simulink library "WBToolboxLibrary"  (R2014b)
settings: Solver=ode45  StartTime=0.0  StopTime=10.0  RelTol=1e-3
undefined symbols (not defined in the file): WBT_modelName, WBT_robotName, WBT_wbiFilename, WBT_wbiList
libraries: simulink x1
(part 1 of 2)
settings Model: CovSaveCumulativeToWorkspaceVar=on  Creator=jorhabib  LastModifiedBy=csartore

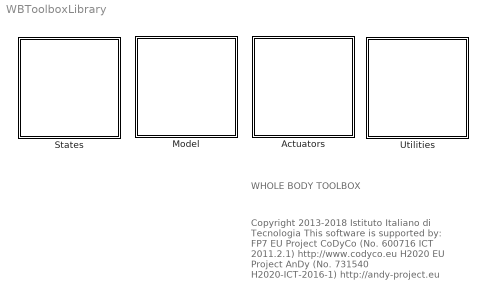
== system WBToolboxLibrary ==
  note: WHOLE BODY TOOLBOX
  note: Copyright 2013-2018 Istituto Italiano di Tecnologia
      |
      | This software is supported by:
      | FP7 EU Project CoDyCo (No. 600716 ICT 2011.2.1) http://www.codyco.eu
      | H2020 EU Project AnDy (No. 731540 H2020-ICT-2016-1) http://andy-project.eu
  Actuators : Subsystem
      mask Display: image(imread('wholeBodyActuators.png'),'center')
  Model : Subsystem
      mask Display: image(imread('wholeBodyModel.png'),'center')
  States : Subsystem
      mask Display: image(imread('wholeBodyStates.png'),'center');
  Utilities : Subsystem
      mask Display: image(imread('utilities.png'))

== system WBToolboxLibrary/Actuators ==
  SetMotorParameters : S-Function  FunctionName=BlockFactory  Parameters='SetMotorParameters','WBToolbox',WBTConfigParameters,configBlockAbsName,readP,readI,readD,pidType,setKTau,kTau,setBemf,bemf  SFunctionDeploymentMode=off  EnableBusSupport=off  mask(SetMotorParameters){pidType=Position, readP=on, readI=off, readD=off, setKTau=off, kTau=[0], setBemf=off, bemf=[0]}
      mask prompts: pidType "PID Type"; readP "Enable P gains input signal"; readI "Enable I gains input signal"; readD "Enable D gains input signal"; setKTau "Set motor constant KTau"; setBemf "Set motor back EMF constant"
      mask help:
      | This block allows to set motor PIDs and constants such as the motor constant and the back EMF.
      |
      | The motor constant and the back EMF are set in the block's mask, and their values are applied during the first simulation loop. The PIDs values are instead set from the input ports.
      |
      | All these vectors should have a size equal to the number of controlled joints specified in the referred Configuration block.
      |
      | At the end of the simulation, the default values are restored.
      mask init:
      | % WBBlock Initialization
      | % ======================
      | 
      | try
      |     [configBlockAbsName, WBTConfig] = WBToolbox.BlockInitialization(gcb, gcs);
      |     
      |     WBTConfigParameters = WBTConfig.getSimulinkParameters;
      |     clear WBTConfig;
      | catch
      | end
      | 
      | % The booleans of the checkboxes always create problems
      | readP = uint8(readP);
      | readI = uint8(readI);
      | readD = uint8(readD);
      mask TypeOptions pidType: Position | Torque
      mask Callback pidType:
      | % Get the mask parameter values. This is a cell
      | %   array of strings.
      | maskStr = get_param(gcb,'pidType');
      | 
      | switch maskStr
      |     case 'Position'
      |         set_param(gcb,'BackgroundColor', '[0.5137, 0.8510, 0.6706, 1.0]');
      |     case 'Position Direct'
      |         set_param(gcb,'BackgroundColor', '[0.3922, 0.7882, 0.3451, 1.0]');
      |     case 'Velocity'
      |         set_param(gcb,'BackgroundColor', '[0.5137, 0.6745, 1.0000, 1.0]');
      |     case 'Torque'
      |         set_param(gcb,'BackgroundColor', '[0.8275, 0.5765, 0.6039, 1.0]');
      |     otherwise
      |         error('PID Type not recognized');
      | end
      | 
      | clear  maskStr
      mask Callback setKTau:
      | h = Simulink.Mask.get(gcb);
      | setKTauValue = get_param(gcb,'setKTau');
      | 
      | if ~strcmp(setKTauValue,'on')
      |     h.Parameters(6).Enabled = 'off';
      | else
      |     h.Parameters(6).Enabled = 'on';
      | end
      | 
      | clear h setKTauValue
      mask Callback setBemf:
      | h = Simulink.Mask.get(gcb);
      | setBemfValue = get_param(gcb,'setBemf');
      | 
      | if ~strcmp(setBemfValue,'on')
      |     h.Parameters(8).Enabled = 'off';
      | else
      |     h.Parameters(8).Enabled = 'on';
      | end
      | 
      | clear h setBemfValue
      mask DialogControl Control2 Prompt: Toggle Config Block Highlighting
      mask DialogControl Control2 Callback:
      | [configBlock, ~] = WBToolbox.BlockInitialization(gcb, gcs);
      | 
      | try
      |     if (strcmp(get_param(configBlock,'HiliteAncestors'),'none'))
      |         hilite_system(configBlock,'find');
      |     else
      |         hilite_system(configBlock,'none');
      |     end
      | catch
      |     error('[%s:ShowConfigBlock:Callback] Failed to process config block name: %s',gcb,configBlock);
      | end
      | 
      | clear configBlock
      mask Display:
      | fprintf('Motor Parameters\n(%s)',pidType);
      | 
      | numPorts = 0;
      | 
      | if readP
      |     numPorts = numPorts + 1;
      |     port_label('input',numPorts,'P')
      | end
      | 
      | if readI
      |     numPorts = numPorts + 1;
      |     port_label('input',numPorts,'I')
      | end
      | 
      | if readD
      |     numPorts = numPorts + 1;
      |     port_label('input',numPorts,'D')
      | end
  SetMotorReferences : Subsystem  mask(SetMotorReferences){controlType=Current}
      mask prompts: controlType "Control Mode"
      mask help:
      | This block sets motor references. The type of control mode is specified as a parameter in the block.
      |
      | Assuming N as the number of motors (usually equal to internal DoFs):
      |
      | Input:
      |   - References: Vector of size N, representing the references to be sent to the robot controlled motors.
      |
      | Parameters:
      |   - Control Mode: The control mode. Choose one of the supplied mode.
      |
      | Unit of measurement:
      |   - PWM  [-100, 100]% Duty cycle
      |   - Current [A]
      |   - Back EMF
      |   - Torque Constant
      mask init:
      | refSpeed = 0;
      | 
      | % WBBlock Initialization
      | % ======================
      | 
      | try
      |     [configBlockAbsName, WBTConfig] = WBToolbox.BlockInitialization(gcb, gcs);
      |     
      |     WBTConfigParameters = WBTConfig.getSimulinkParameters;
      |     clear WBTConfig;
      | catch
      | end
      mask TypeOptions controlType: PWM | Current | Back EMF | Torque Constant
      mask Callback controlType:
      | % Get the mask parameter values. This is a cell
      | %   array of strings.
      | 
      | maskStr = get_param(gcb,'controlType');
      | 
      | switch maskStr
      |     case 'PWM'
      |         set_param(gcb,'BackgroundColor', '[1, 1, 1, 1.0]');
      |     case 'Current'
      |         set_param(gcb,'BackgroundColor', '[0.96, 0.77, 0.46, 1.0]');
      |     case 'Back EMF'
      |         set_param(gcb,'BackgroundColor', '[0.8, 0.4, 1.0, 1.0]');
      |     case 'Torque Constant'
      |         set_param(gcb,'BackgroundColor', '[0.8, 1.0, 0.4, 1.0]');
      |     otherwise
      |         error('Control Type not recognized.')
      | end
      | 
      | clear  maskStr
      mask DialogControl toggleHighlighting Prompt: Toggle Config Block Highlighting
      mask DialogControl toggleHighlighting Callback:
      | [configBlock, ~] = WBToolbox.BlockInitialization(gcb, gcs);
      | 
      | try
      |     if (strcmp(get_param(configBlock,'HiliteAncestors'),'none'))
      |         hilite_system(configBlock,'find');
      |     else
      |         hilite_system(configBlock,'none');
      |     end
      | catch
      |     error('[%s:ShowConfigBlock:Callback] Failed to process config block name: %s',gcb,configBlock);
      | end
      | 
      | clear configBlock
      mask Display:
      | disp(get_param(gcb,'controlType'))
      | %port_label('input',1,'References')
  SetReferences : Subsystem  mask(SetReferences){controlType=Position, refSpeed=10*(pi/180), refAcceleration=1000000*(pi/180)}
      mask prompts: controlType "Control Mode"; refSpeed "Reference Speed"; refAcceleration "Reference Velocity"
      mask help:
      | This block sets the references for the robot actuators.
      | The type of control mode is specified as a parameter in the block.
      |
      | Assuming DoFs is the number of internal degrees of freedom configured in the associated Config block:
      |
      | Input:
      |   - References: Vector of size DoFs, representing the references to be sent to the robot controlled joints.
      |   - Reference Speed (Position): Set the reference speed in rad/s used by the trajectory generator of the IPositionControl interface
      |   - Reference Acceleration (Velocity): Set the reference speed in rad/s/s used by the trajectory generator of the IVelocityControl interface
      |
      | Parameters:
      |   - Control Mode: The control mode. Choose one of the supplied mode.
      |
      | Unit of measurement:
      | - Position [rad]
      | - Velocity [rad/s]
      | - Acceleration [rad/s/s]
      | - Torque [Nm]
      mask init:
      | if (strcmp(controlType,'Position'))
      |     refTrajectory = refSpeed;
      | elseif (strcmp(controlType,'Velocity'))
      |     refTrajectory = refAcceleration;
      | else
      |     refTrajectory = 0;
      | end
      | 
      | % WBBlock Initialization
      | % ======================
      | 
      | try
      |     [configBlockAbsName, WBTConfig] = WBToolbox.BlockInitialization(gcb, gcs);
      |     
      |     WBTConfigParameters = WBTConfig.getSimulinkParameters;
      |     clear WBTConfig;
      | catch
      | end
      mask TypeOptions controlType: Position | Position Direct | Velocity | Torque
      mask Callback controlType:
      | % Get the mask parameter values. This is a cell
      | %   array of strings.
      | 
      | maskStr = get_param(gcb,'controlType');
      | 
      | switch maskStr
      |     case 'Position'
      |         set_param(gcb,'BackgroundColor', '[0.5137, 0.8510, 0.6706, 1.0]');
      |         set_param(gcb,'MaskVisibilities', {'on';'on';'off'});
      |     case 'Position Direct'
      |         set_param(gcb,'BackgroundColor', '[0.3922, 0.7882, 0.3451, 1.0]');
      |         set_param(gcb,'MaskVisibilities', {'on';'off';'off'});
      |     case 'Velocity'
      |         set_param(gcb,'BackgroundColor', '[0.5137, 0.6745, 1.0000, 1.0]');
      |         set_param(gcb,'MaskVisibilities', {'on';'off';'on'});
      |     case 'Torque'
      |         set_param(gcb,'BackgroundColor', '[0.8275, 0.5765, 0.6039, 1.0]');
      |         set_param(gcb,'MaskVisibilities', {'on';'off';'off'});
      |     otherwise
      |         error('Control Type not recognized.')
      | end
      | 
      | clear  maskStr
      mask DialogControl toggleHighlighting Prompt: Toggle Config Block Highlighting
      mask DialogControl toggleHighlighting Callback:
      | [configBlock, ~] = WBToolbox.BlockInitialization(gcb, gcs);
      | 
      | try
      |     if (strcmp(get_param(configBlock,'HiliteAncestors'),'none'))
      |         hilite_system(configBlock,'find');
      |     else
      |         hilite_system(configBlock,'none');
      |     end
      | catch
      |     error('[%s:ShowConfigBlock:Callback] Failed to process config block name: %s',gcb,configBlock);
      | end
      | 
      | clear configBlock
      mask Display:
      | disp(get_param(gcb,'controlType'))
      | %port_label('input',1,'References')

== system WBToolboxLibrary/Model ==
  Dynamics : Subsystem
      mask Display: image(imread('Dynamics.png'))
  Jacobians : Subsystem
      mask Display: image(imread('jacobian.png'))
  Kinematics : Subsystem
      mask Display: image(imread('forwardKinematics.png'))

== system WBToolboxLibrary/States ==
  GetLimits : Subsystem  mask(GetLimits){limitsSource=ControlBoard, limitsType=Position}
      mask prompts: limitsSource "Limits Source"; limitsType "Limits Type"
      mask help:
      | This block provides the joint limits gathering data from either the Robot's Control Board or URDF model.
      |
      | Output:
      |   - Max: 1xDoFs vector containing the maximum limit
      |   - Min:  1xDoFs vector containing the maximum limit
      |
      | Unit of measurement:
      |   - Position: rad
      |   - Velocity: rad/sec
      mask init:
      | % WBBlock Initialization
      | % ======================
      | 
      | try
      |     [configBlockAbsName, WBTConfig] = WBToolbox.BlockInitialization(gcb, gcs);
      |     
      |     WBTConfigParameters = WBTConfig.getSimulinkParameters;
      |     clear WBTConfig;
      | catch
      | end
      | 
      | % GetLimits Initialization
      | % =========================
      | 
      | sourceLimit = get_param(gcb,'limitsSource');
      | typeLimit = get_param(gcb,'limitsType');
      | notifyError = false;
      | 
      | switch sourceLimit
      |     case 'ControlBoard'
      |         switch typeLimit
      |             case 'Position'
      |                 limitsType = 'ControlBoardPosition';
      |             case 'Velocity'
      |                 limitsType = 'ControlBoardVelocity';
      |             otherwise
      |                 notifyError = true;
      |         end
      |     case 'URDF'
      |         switch typeLimit
      |             case 'Position'
      |                 limitsType = 'ModelPosition';
      |             otherwise
      |                 notifyError = true;
      |         end
      | end
      | 
      | if notifyError
      |     error('Limit Type not recognized');
      | end
      | 
      | clear sourceLimit typeLimit notifyError
      mask TypeOptions limitsSource: ControlBoard | URDF
      mask Callback limitsSource:
      | sourceLimit = get_param(gcb,'limitsSource');
      | blockParameters = Simulink.Mask.get(gcb).Parameters;
      | limitsTypeBlockParam = blockParameters(2);
      | 
      | switch sourceLimit
      |     case 'ControlBoard'
      |         limitsTypeBlockParam.TypeOptions = {'Position','Velocity'};
      |         %limitsTypeBlockParam.Value = limitsTypeBlockParam.TypeOptions{1};
      |     case 'URDF'
      |         limitsTypeBlockParam.TypeOptions = {'Position'};
      |         %limitsTypeBlockParam.Value = limitsTypeBlockParam.TypeOptions{1};
      |     otherwise
      |         error('Limit Source not recognized');
      | end
      | 
      | clear sourceLimit blockParameters limitsTypeBlockParam
      mask TypeOptions limitsType: Position | Velocity
      mask Callback limitsType:
      | % Get the mask parameter values. This is a cell array of strings.
      | %
      | maskStr = get_param(gcb,'limitsType');
      | if strcmp(maskStr, 'Position')
      |     set_param(gcb,'BackgroundColor', '[0.5137, 0.8510, 0.6706, 1.0]');
      | elseif strcmp(maskStr, 'Velocity')
      |     set_param(gcb,'BackgroundColor', '[0.5137, 0.6745, 1.0000, 1.0]');
      | elseif strcmp(maskStr, 'Acceleration')
      |     set_param(gcb,'BackgroundColor', '[0.9255, 0.8706, 0.1333, 1.0]');
      | elseif strcmp(maskStr, 'Torque')
      |     set_param(gcb,'BackgroundColor', '[0.8275, 0.5765, 0.6039, 1.0]');
      | end
      | clear  maskStr
      mask DialogControl toggleHighlighting Prompt: Toggle Config Block Highlighting
      mask DialogControl toggleHighlighting Callback:
      | [configBlock, ~] = WBToolbox.BlockInitialization(gcb, gcs);
      | 
      | try
      |     if (strcmp(get_param(configBlock,'HiliteAncestors'),'none'))
      |         hilite_system(configBlock,'find');
      |     else
      |         hilite_system(configBlock,'none');
      |     end
      | catch
      |     error('[%s:ShowConfigBlock:Callback] Failed to process config block name: %s',gcb,configBlock);
      | end
      | 
      | clear configBlock
      mask Display:
      | fprintf('%s\n(%s)',get_param(gcb,'limitsType'),get_param(gcb,'limitsSource'))
      | 
      | port_label('output',1,'Min')
      | port_label('output',2,'Max')
  GetMeasurement : Subsystem  mask(GetMeasurement){measuredType=Joints Position}
      mask prompts: measuredType "Estimate Type"
      mask help:
      | This block gathers the measurement of the specified type.
      |
      | Assuming DoFs is the number of degrees of freedom of the robot,
      |
      | Output:
      |   - References: Vector of size DoFs, representing the requested measurement.
      |
      | Parameters:
      |   - Control Mode: The control mode. Choose one of the supplied mode.
      |
      | Unit of measurement:
      |   - Position: rad
      |   - Velocity: rad/sec
      |   - Acceleration: rad/sec/sec
      |   - Torque: Nm
      mask init:
      | % WBBlock Initialization
      | % ======================
      | 
      | try
      |     [configBlockAbsName, WBTConfig] = WBToolbox.BlockInitialization(gcb, gcs);
      |     
      |     WBTConfigParameters = WBTConfig.getSimulinkParameters;
      |     clear WBTConfig;
      | catch
      | end
      mask TypeOptions measuredType: Joints Position | Joints Velocity | Joints Acceleration | Joints Torque
      mask Callback measuredType:
      | % Get the mask parameter values. This is a cell
      | %   array of strings.
      | 
      | maskStr = get_param(gcb,'measuredType');
      | if strcmp(maskStr, 'Joints Position')
      |     set_param(gcb,'BackgroundColor', '[0.5137, 0.8510, 0.6706, 1.0]');
      | elseif strcmp(maskStr, 'Joints Velocity')
      |     set_param(gcb,'BackgroundColor', '[0.5137, 0.6745, 1.0000, 1.0]');
      | elseif strcmp(maskStr, 'Joints Acceleration')
      |     set_param(gcb,'BackgroundColor', '[0.9255, 0.8706, 0.1333, 1.0]');
      | elseif strcmp(maskStr, 'Joints Torque')
      |     set_param(gcb,'BackgroundColor', '[0.8275, 0.5765, 0.6039, 1.0]');
      | end
      | clear  maskStr
      mask DialogControl toggleHighlighting Prompt: Toggle Config Block Highlighting
      mask DialogControl toggleHighlighting Callback:
      | [configBlock, ~] = WBToolbox.BlockInitialization(gcb, gcs);
      | 
      | try
      |     if (strcmp(get_param(configBlock,'HiliteAncestors'),'none'))
      |         hilite_system(configBlock,'find');
      |     else
      |         hilite_system(configBlock,'none');
      |     end
      | catch
      |     error('[%s:ShowConfigBlock:Callback] Failed to process config block name: %s',gcb,configBlock);
      | end
      | 
      | clear configBlock
      mask Display: port_label('output', 1, get_param(gcb,'measuredType'))
  GetMotorMeasurement : Subsystem  mask(GetMeasurement){measuredType=Motor Current}
      mask prompts: measuredType "Estimate Type"
      mask help:
      | This block gathers the measurement of the specified type.
      |
      | Assuming DoFs is the number of degrees of freedom of the robot,
      |
      | Output:
      |   - References: Vector of size DoFs, representing the requested measurement.
      |
      | Parameters:
      |   - Control Mode: The control mode. Choose one of the supplied mode.
      |
      | Unit of measurement:
      |   - PWM: duty cycle expressed as percentage [-100, 100]%
      |   - Current: values in Ampere
      mask init: same as WBToolboxLibrary/States/GetMeasurement
      mask TypeOptions measuredType: Motor Position | Motor Velocity | Motor Acceleration | Motor PWM | Motor Current | Motor Back EMF | Motor Torque Constant
      mask Callback measuredType:
      | maskStr = get_param(gcb,'measuredType');
      | 
      | switch maskStr
      |     case 'Motor Position'
      |         set_param(gcb,'BackgroundColor', '[0.5137, 0.8510, 0.6706, 1.0]');
      |     case 'Motor Velocity'
      |         set_param(gcb,'BackgroundColor', '[0.5137, 0.6745, 1.0000, 1.0]');
      |     case 'Motor Acceleration'
      |         set_param(gcb,'BackgroundColor', '[0.9255, 0.8706, 0.1333, 1.0]');
      |     case 'Motor PWM'
      |         set_param(gcb,'BackgroundColor', '[1, 1, 1, 1.0]');
      |     case 'Motor Current'
      |         set_param(gcb,'BackgroundColor', '[0.96, 0.77, 0.46, 1.0]');
      |     case 'Motor Back EMF'
      |         set_param(gcb,'BackgroundColor', '[0.8, 0.4, 1.0, 1.0]');
      |     case 'Motor Torque Constant'
      |         set_param(gcb,'BackgroundColor', '[0.8, 1.0, 0.4, 1.0]');
      |     otherwise
      |         error('Control Type not recognized.')
      | end
      | 
      | clear maskStr
      mask DialogControl toggleHighlighting Prompt: Toggle Config Block Highlighting
      mask DialogControl toggleHighlighting Callback:
      | [configBlock, ~] = WBToolbox.BlockInitialization(gcb, gcs);
      | 
      | try
      |     if (strcmp(get_param(configBlock,'HiliteAncestors'),'none'))
      |         hilite_system(configBlock,'find');
      |     else
      |         hilite_system(configBlock,'none');
      |     end
      | catch
      |     error('[%s:ShowConfigBlock:Callback] Failed to process config block name: %s',gcb,configBlock);
      | end
      | 
      | clear configBlock
      mask Display: port_label('output', 1, get_param(gcb,'measuredType'))

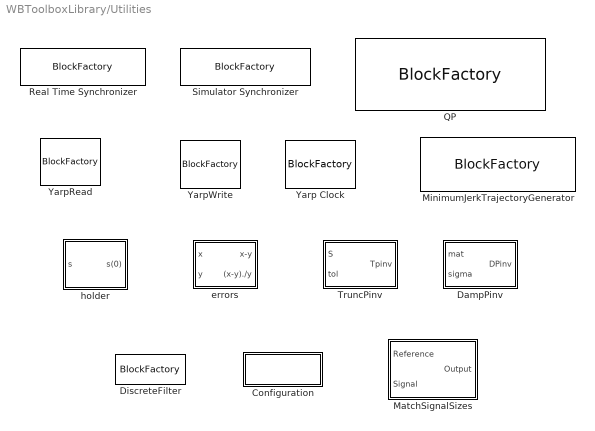
== system WBToolboxLibrary/Utilities ==
  Configuration : Subsystem  InitFcn=|  mask{ConfigSource=Mask, ConfigObject='WBTConfigRobot', RobotName='icubSim', UrdfFile='model.urdf', ControlledJoints={'l_elbow','l_shoulder_pitch','torso_roll'}, ControlBoardsNames={'left_arm','right_arm','torso'}, LocalName='WBT', GravityVector=[0,0,-9.81]}
      | source = get_param(gcb,'ConfigSource');
      | 
      | if strcmp(source, 'Workspace')
      |     object = get_param(gcb,'ConfigObject');
      |     WBToolbox.ConfigurationToMask(gcb, object);
      | end
      | 
      | WBToolbox.MaskToConfiguration(gcb);
      | 
      | clear object source
      mask prompts: ConfigSource "Configuration from"; ConfigObject "Name of the object"; RobotName "Robot Name"; UrdfFile "Urdf File"; ControlledJoints "Controlled Joints"; ControlBoardsNames "Control Boards Names"; LocalName "Local Name"; GravityVector "Gravity Vector"
      mask TypeOptions ConfigSource: Workspace | Mask
      mask Callback ConfigSource:
      | % Get the Workspace/Mask menu
      | h = Simulink.Mask.get(gcb);
      | currentConfigSource = get_param(gcb,'ConfigSource');
      | 
      | if strcmp(currentConfigSource,'Workspace')
      |     % Switch the visibility of the GUI elements
      |     set_param(gcb,'MaskVisibilities',{'on';'on';'on';'on';'on';'on';'on';'on';});
      |     h.Parameters(3).ReadOnly = 'on';
      |     h.Parameters(4).ReadOnly = 'on';
      |     h.Parameters(5).ReadOnly = 'on';
      |     h.Parameters(6).ReadOnly = 'on';
      |     h.Parameters(7).ReadOnly = 'on';
      |     h.Parameters(8).ReadOnly = 'on';
      | 
      |     % Parse the object inserted in the ConfigObject field
      |     currentConfigObject = get_param(gcb,'ConfigObject');
      |     WBToolbox.ConfigurationToMask(gcb,currentConfigObject);
      |     clear currentConfigObject;
      | elseif strcmp(currentConfigSource,'Mask')
      |     % Switch the visibility of the GUI elements
      |     set_param(gcb,'MaskVisibilities',{'on';'off';'on';'on';'on';'on';'on';'on';});
      |     h.Parameters(3).ReadOnly = 'off';
      |     h.Parameters(4).ReadOnly = 'off';
      |     h.Parameters(5).ReadOnly = 'off';
      |     h.Parameters(6).ReadOnly = 'off';
      |     h.Parameters(7).ReadOnly = 'off';
      |     h.Parameters(8).ReadOnly = 'off';
      |     h.Parameters(3).Enabled = 'on';
      |     h.Parameters(4).Enabled = 'on';
      |     h.Parameters(5).Enabled = 'on';
      |     h.Parameters(6).Enabled = 'on';
      |     h.Parameters(7).Enabled = 'on';
      |     h.Parameters(8).Enabled = 'on';
      | end
      | 
      | clear h currentConfigSource
      mask Callback ConfigObject:
      | % This code get called whatsoever
      | if strcmp(char(get_param(gcb,'ConfigSource')),'Mask')
      |     return
      | end
      | 
      | % Parse the object inserted in the ConfigObject field
      | currentConfigObject = get_param(gcb,'ConfigObject');
      | WBToolbox.ConfigurationToMask(gcb,currentConfigObject);
      | 
      | clear currentConfigObject;
      mask Display: disp('Config')
  DampPinv : Subsystem  mask{tol=1e-4}
      mask prompts: tol "Tolerance"
  DiscreteFilter : S-Function  FunctionName=BlockFactory  Parameters='DiscreteFilter','WBToolbox',filterDataStruct  SFunctionDeploymentMode=off  EnableBusSupport=off  mask(DiscreteFilter){filterType=Generic, numCoeffs=[0], denCoeffs=[0], Fc=0, Ts=0, orderMedianFilter=0, initStatus=off, y0=[0], u0=[0]}
      mask prompts: filterType "Type of the filter"; numCoeffs "Numerator Coefficients*"; denCoeffs "Denominator Coefficients*"; Fc "Cut Frequency (Hz)"; Ts "Sampling time (s)"; orderMedianFilter "Order"; initStatus "Define initial conditions"; y0 "Output y0"; u0 "Input u0"
      mask help: This block wraps the Filter, FirstOrderLowPassFilter, and MedianFilter from iCub::ctrl.
      mask init:
      | filterDataStruct = struct;
      | filterDataStruct.Fc = Fc;
      | filterDataStruct.Ts = Ts;
      | filterDataStruct.MedianOrder = orderMedianFilter;
      | filterDataStruct.FilterType = filterType;
      | filterDataStruct.NumCoeffs = numCoeffs;
      | filterDataStruct.DenCoeffs = denCoeffs;
      | filterDataStruct.y0 = y0;
      | filterDataStruct.u0 = u0;
      | filterDataStruct.InitStatus = uint8(initStatus);
      mask TypeOptions filterType: Generic | FirstOrderLowPassFilter | MedianFilter
      mask Callback filterType:
      | % From: https://it.mathworks.com/help/simulink/slref/simulink.mask-class.html
      | filterType = get_param(gcb, 'filterType');
      | initStatus = get_param(gcb, 'initStatus');
      | p = Simulink.Mask.get(gcbh);
      | howToCoeffs = p.getDialogControl('howToCoeffs');
      | 
      | %set_param(gcb, 'initStatus','off');
      | if (strcmp(initStatus,'on'))
      |     vis_init = 'on';
      | else
      |     vis_init = 'off';
      | end
      | 
      | if(strcmp(filterType, 'Generic'))
      |     set_param(gcb, 'MaskVisibilities',{'on','on','on','off','off','off','on',vis_init,vis_init});
      |     howToCoeffs.Visible = 'on';
      | elseif(strcmp(filterType, 'FirstOrderLowPassFilter'))
      |     set_param(gcb, 'MaskVisibilities',{'on','off','off','on','on','off','on',vis_init,'off'});
      |     howToCoeffs.Visible = 'off';
      | elseif(strcmp(filterType, 'MedianFilter'))
      |     set_param(gcb, 'MaskVisibilities',{'on','off','off','off','off','on','on',vis_init,'off'});
      |     howToCoeffs.Visible = 'off';
      | end
      | 
      | clear filterType initStatus p howToCoeffs vis_init;
      mask Callback initStatus:
      | initStatus   = get_param(gcb, 'initStatus');
      | visibilities = get_param(gcb, 'MaskVisibilities');
      | filterType   = get_param(gcb, 'filterType');
      | 
      | if (strcmp(initStatus,'off'))
      |     visibilities{8} = 'off';
      |     visibilities{9} = 'off';
      | elseif (strcmp(initStatus,'on'))
      |     visibilities{8} = 'on';
      |     if (strcmp(filterType,'Generic'))
      |         visibilities{9} = 'on';
      |     end
      | end
      | 
      | set_param(gcb, 'MaskVisibilities', visibilities);
      | 
      | clear initStatus visibilities filterType;
      mask DialogControl howToCoeffs Prompt: * The coefficients are ordered in increasing power of z^-1
      mask Display: disp('Filter')
  MatchSignalSizes : Subsystem  mask(MatchSignalSizes){}
      mask help:
      | It can happen on particular cases that the Simulink engine cannot propagate the right sizes from blocks of the toolbox. If you encounter such problems you can try using this blocks which introducing a minimal overhead assigns to input Signal the same size of input Reference and outputs Signal.
      |
      | Currently it supports only 1D vectors.
      mask Display:
      | port_label('input', 1, 'Reference')
      | port_label('input', 2, 'Signal')
      | port_label('output', 1, 'Signal')
  MinimumJerkTrajectoryGenerator : S-Function  FunctionName=BlockFactory  Parameters='MinimumJerkTrajectoryGenerator','WBToolbox',sampleTime,settlingTime,firstDerivatives,secondDerivatives,explicitInitialValue,externalSettlingTime,resetOnSettlingTime  SFunctionDeploymentMode=off  EnableBusSupport=off  mask(MinimumJerkTrajectoryGenerator){externalSettlingTime=off, settlingTime=3, sampleTime=0.01, resetOnSettlingTime=off, firstDerivatives=on, secondDerivatives=on, explicitInitialValue=off}
      mask prompts: externalSettlingTime "External Settling Time"; settlingTime "Settling Time"; sampleTime "Sample Time"; resetOnSettlingTime "Reset on Settling Time Changes"; firstDerivatives "Output First Derivative"; secondDerivatives "Output Second Derivative"; explicitInitialValue "Explicit Initial Value"
      mask help:
      | This block wraps the minJerkTrajGen class from iCub::ctrl::minJerkTrajGen.
      |
      | The Minimum Jerk Trajectory Generator is approximated using a 3rd order LTI dynamical system (for more details see [1]).
      |
      | Position, velocity and acceleration trajectories are computed.
      |
      | The main advantage with respect to the standard polynomial form is that if the reference value yd changes there is no need to recompute the filter coefficients.
      |
      | [1]
      | Pattacini, U.; Nori, F.; Natale, L.; Metta, G.; Sandini, G.
      | "An experimental evaluation of a novel minimum-jerk cartesian controller for humanoid robots"
      | Intelligent Robots and Systems (IROS), 2010
      | IEEE/RSJ International Conference on , vol., no., pp.1668-1674, 18-22 Oct. 2010
      | doi: 10.1109/IROS.2010.5650851
      | URL: http://ieeexplore.ieee.org/stamp/stamp.jsp?tp=&arnumber=5650851&isnumber=5648787
      mask Callback externalSettlingTime:
      | externalSettlingTime = get_param(gcb, 'externalSettlingTime');
      | visibility = get_param(gcb, 'MaskVisibilities');
      | if(strcmp(externalSettlingTime, 'on'))
      |     visibility{2} = 'off';
      |     visibility{4} = 'on';
      | else
      |     visibility{2} = 'on';
      |     visibility{4} = 'off';
      | end
      | set_param(gcb, 'MaskVisibilities',visibility);
      | clear externalSettlingTime
      mask Display:
      | firstDer = get_param(gcb, 'firstDerivatives');
      | secondDer = get_param(gcb, 'secondDerivatives');
      | initialValues = get_param(gcb, 'explicitInitialValue');
      | externalSettlingTimeParam = get_param(gcb, 'externalSettlingTime');
      | 
      | %Inputs
      | portIndex = 2;
      | port_label('input', 1, 'Reference')
      | if(strcmp(initialValues, 'on'))
      |     port_label('input', portIndex, 'Initial Value')
      |     portIndex = portIndex + 1;
      | end
      | 
      | if(strcmp(externalSettlingTimeParam, 'on'))
      |     port_label('input', portIndex, 'Settling Time')
      |     portIndex = portIndex + 1;
      | end
      | 
      | %Outputs
      | port_label('output', 1, 'Signal')
      | secondDerPortIndex = 2;
      | if(strcmp(firstDer, 'on'))
      |     port_label('output', 2, 'First Derivative')
      |     secondDerPortIndex = secondDerPortIndex + 1;
      | end
      | if(strcmp(secondDer, 'on'))
      |     port_label('output', secondDerPortIndex, 'Second Derivative')
      | end
  QP : S-Function  FunctionName=BlockFactory  Parameters='QpOases','WBToolbox',lbA,ubA,lb,ub,computeObjVal,stopIfFails  SFunctionDeploymentMode=off  EnableBusSupport=off  mask(QP){lbA=off, ubA=on, lb=off, ub=off, computeObjVal=off, stopIfFails=off}
      mask prompts: lbA "Accept constraints lower bound input (lbA)"; ubA "Accept constraints upper bound input (ubA)"; lb "Accept lower bound input (lb)"; ub "Accept upper bound input (ub)"; computeObjVal "Output the value of the objective function"; stopIfFails "Stop the simulation if the solver fails"
      mask help:
      | This block solves a QP problem using the qpOASES library:
      |
      | x = argmin 0.5 * x' * H * x + c' * x
      |
      | s.t.
      |
      | lbA <= Ax <= ubA
      | lb <= x <= ub
      mask Display:
      | disp('QP')
      | 
      | port_label('output', 1, 'PrimalSolution')
      | port_label('output', 2, 'Status')
      | 
      | if (computeObjVal)
      |     port_label('output', 3, 'Obj func value')
      | end
      | 
      | port_label('input', 1, 'H');
      | port_label('input', 2, 'g');
      | 
      | inputPortNumber = 2;
      | 
      | if (lbA || ubA)
      |     inputPortNumber = 3;
      |     port_label('input', 3, 'A');
      | end
      | 
      | if (lbA)
      |     inputPortNumber = inputPortNumber + 1;
      |     port_label('input', inputPortNumber, 'lbA');
      | end
      | if (ubA)
      |     inputPortNumber = inputPortNumber + 1;
      |     port_label('input', inputPortNumber, 'ubA');
      | end
      | if (lb)
      |     inputPortNumber = inputPortNumber + 1;
      |     port_label('input', inputPortNumber, 'lb');
      | end
      | if (ub)
      |     inputPortNumber = inputPortNumber + 1;
      |     port_label('input', inputPortNumber, 'ub');
      | end
  Real Time Synchronizer : S-Function  FunctionName=BlockFactory  Parameters='RealTimeSynchronizer','WBToolbox',period  SFunctionDeploymentMode=off  EnableBusSupport=off  mask(Real Time Synchronizer){period=0.01}
      mask prompts: period "Controller Period (in seconds)"
      mask help:
      | This block slows down the simulation trying to match the period specified
      | as parameter (in seconds).
      | The bigger the period the more probable
      | is that Simulink can remain synched with it.
      mask Display: disp('Real Time Synchronizer')
  Simulator Synchronizer : S-Function  FunctionName=BlockFactory  Parameters='SimulatorSynchronizer','WBToolbox',period, serverPortName, clientPortName  SFunctionDeploymentMode=off  EnableBusSupport=off  mask(Simulator Synchronizer){period=0.01, serverPortName='/clock/rpc', clientPortName='/WBT_synchronizer/rpc:o'}
      mask prompts: period "Controller Period (in seconds)"; serverPortName "Server Port Name"; clientPortName "Client Port Name"
      mask help:
      | This block synchronizes with the external simulation on a simulator
      | (only Gazebo is supported at the moment).
      mask Display: disp('Simulator Synchronizer')
  TruncPinv : Subsystem  mask{tol=1e-4}
      mask prompts: tol "Tolerance"
  Yarp Clock : S-Function  FunctionName=BlockFactory  Parameters='YarpClock','WBToolbox'  SFunctionDeploymentMode=off  EnableBusSupport=off  mask(YARP Clock){}
      mask help:
      | This block outputs the current YARP Time.
      | In a nutshell, this block outputs the equivalent of the C++ function call yarp::os::Time::now()
      mask Display: disp('YARP Time')
  YarpRead : S-Function  FunctionName=BlockFactory  Parameters='YarpRead','WBToolbox',portName,signalSize,blocking,timestamp,autoconnect,errorOnConnection,timeout  SFunctionDeploymentMode=off  EnableBusSupport=off  mask(YARP Read){portName='/portname', signalSize=1, timeout=0.5, blocking=off, timestamp=on, autoconnect=on, errorOnConnection=on}
      mask prompts: portName "Source Port Name"; signalSize "Port Size"; blocking "Blocking Read"; timestamp "Read Timestamp"; errorOnConnection "Error on missing connection"
      mask help:
      | This block behaves as the command 'yarp read'.
      |
      | By default it has the option 'Autoconnect' active, which means that the user can only specify the name of the port ('Source Port Name') from which readings are desired, along with the size of the expected data (e.g. 3 when reading the torso state).
      |
      | When the user unchecks 'Autoconnect', 'Opened Port Name' field shows up and it corresponds to the name of the port the block will create. No autoconnection is performed, and the output will be always zero until the user connects it to some other port from command line using 'yarp connect [from] [dest]'.
      |
      | When 'Autoconnect' is off, an additional output called 'signal' is added to the block. It outputs 1 if the port has received at least one sample, or 0 otherwise.
      mask init:
      | % Solve error in string parsing. Force the type.
      | portName = char(portName);
      mask Callback blocking:
      | blocking_val = get_param(gcb, 'blocking');
      | mask_visibility = get_param(gcb, 'MaskVisibilities');
      | 
      | if(strcmp(blocking_val, 'on'))
      |     mask_visibility{3} = 'on';
      |     set_param(gcb, 'MaskVisibilities', mask_visibility);
      | else
      |     mask_visibility{3} = 'off';
      |     set_param(gcb, 'MaskVisibilities', mask_visibility);
      | end
      | 
      | clear blocking_val mask_visibility
      mask Callback autoconnect:
      | autoconnect_val = get_param(gcb, 'Autoconnect');
      | prompt_string = get_param(gcb, 'MaskPrompts');
      | mask_visibilities = get_param(gcb, 'MaskVisibilities');
      | 
      | if(strcmp(autoconnect_val, 'on'))
      |     prompt_string{1} = 'Source Port Name';
      |     mask_visibilities{7} = 'on';
      |     set_param(gcb, 'MaskVisibilities',mask_visibilities);
      | else
      |     prompt_string{1} = 'Opened Port Name';
      |     mask_visibilities{7} = 'off';
      |     set_param(gcb, 'MaskVisibilities',mask_visibilities);
      | end
      | set_param(gcb, 'MaskPrompts', prompt_string);
      | clear autoconnect_val prompt_string mask_visibilities
      mask Display:
      | port_label('output', 1, 'signal');
      | portNumber = 1;
      | if (timestamp)
      |     portNumber = portNumber + 1;
      |     port_label('output', portNumber, 'timestamp');
      | end
      | 
      | if (~autoconnect)
      |     portNumber = portNumber + 1;
      |     port_label('output', portNumber, 'status');
      | end
  YarpWrite : S-Function  FunctionName=BlockFactory  Parameters='YarpWrite','WBToolbox',portName,autoconnect,errorOnConnection  SFunctionDeploymentMode=off  EnableBusSupport=off  mask(YARP Write){portName='/portname', autoconnect=off, errorOnConnection=on}
      mask prompts: portName "Opened Port Name"; errorOnConnection "Error on missing connection"
      mask help:
      | This block behaves as the command 'yarp write'.
      |
      | By default this block opens a port names as the "Opened Port Name" parameter
      | and stream the input signal to that port.
      | If the option "Autoconnect" is specified, the first parameter become the
      | name of the target port to which the data will be stramed,
      | e.g. like "yarp write ... /destinationPort"
      mask Callback autoconnect:
      | autoconnect_val = get_param(gcb, 'Autoconnect');
      | prompt_string = get_param(gcb, 'MaskPrompts');
      | if(strcmp(autoconnect_val, 'on'))
      |     prompt_string{1} = 'Destination Port Name';
      |     set_param(gcb, 'MaskVisibilities',{'on';'on';'on'});
      | else
      |     prompt_string{1} = 'Opened Port Name';
      |     set_param(gcb, 'MaskVisibilities',{'on';'on';'off'});
      | end
      | set_param(gcb, 'MaskPrompts', prompt_string);
      | clear autoconnect_val prompt_string
      mask Display: disp('YarpWrite')
  errors : Subsystem  mask(Errors){}
      mask help:
      | Computes two kinds of errors. The first is just the difference between x
      | and y while the second is the ratio (x-y)/y.
  "holder " : Subsystem  mask(Holder){}
      mask help: This block holds the first input value during the simulation.

== system WBToolboxLibrary/Actuators/SetMotorReferences ==
  References : Inport
  S-Function : S-Function  FunctionName=BlockFactory  Parameters='SetReferences','WBToolbox',WBTConfigParameters,configBlockAbsName,controlType,refSpeed  SFunctionDeploymentMode=off  EnableBusSupport=off
  wires:
  References/1 -> S-Function/1

== system WBToolboxLibrary/Actuators/SetReferences ==
  References : Inport
  S-Function : S-Function  FunctionName=BlockFactory  Parameters='SetReferences','WBToolbox',WBTConfigParameters,configBlockAbsName,controlType,refTrajectory  SFunctionDeploymentMode=off  EnableBusSupport=off
  wires:
  References/1 -> S-Function/1

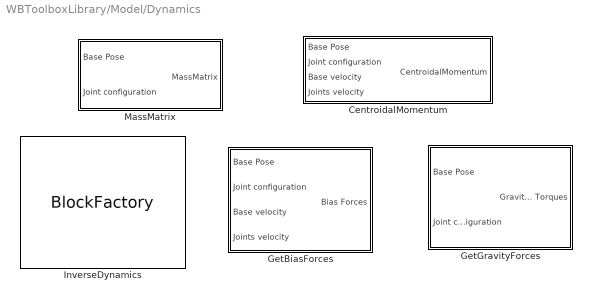
== system WBToolboxLibrary/Model/Dynamics ==
  CentroidalMomentum : Subsystem  mask(CentroidalMomentum){}
      mask help:
      | This block computed the 6 element centroidal momentum, as defined in:
      |
      | "Centroidal dynamics of a humanoid robot" - DE Orin, A Goswami, SH Lee
      | Autonomous Robots 35 (2-3), 161-176
      |
      | Assuming DoFs is the number of internal degrees of freedom of the robot:
      |
      | Input:
      |   - Base pose: 4x4 matrix representing the homogenous transformation between the base frame and the world frame.
      |   - Joint configuration: Vector of size DoFs, representing the configuration of the joints.
      |   - Base velocity: Vector of size 6 representing the linear and angular velocity of the base frame.
      |   - Joints velocity: Vector of size DoFs, representing the velocity of the joints.
      |
      | Output:
      |   - Centroidal Momentum: 6-element vector containg the centroidal momentum (3 value for linear momentum and 3 for angular momentum).
      mask init: same as WBToolboxLibrary/States/GetMeasurement
      mask DialogControl toggleHighlighting Prompt: Toggle Config Block Highlighting
      mask DialogControl toggleHighlighting Callback:
      | [configBlock, ~] = WBToolbox.BlockInitialization(gcb, gcs);
      | 
      | try
      |     if (strcmp(get_param(configBlock,'HiliteAncestors'),'none'))
      |         hilite_system(configBlock,'find');
      |     else
      |         hilite_system(configBlock,'none');
      |     end
      | catch
      |     error('[%s:ShowConfigBlock:Callback] Failed to process config block name: %s',gcb,configBlock);
      | end
      | 
      | clear configBlock
  GetBiasForces : Subsystem  mask(Get Generalized Bias Forces){}
      mask help:
      | This block retrieves the generalied bias forces of the robot.
      |
      | Assuming DoFs is the number of internal degrees of freedom of the robot:
      |
      | Input:
      |   - Base pose: 4x4 matrix representing the homogenous transformation between the base frame and the world frame.
      |   - Joint configuration: Vector of size DoFs, representing the configuration of the joints.
      |   - Base velocity: Vector of size 6 representing the linear and angular velocity of the base frame.
      |   - Joints velocity: Vector of size DoFs, representing the velocity of the joints.
      |
      | Output:
      |   - Bias Forces: a Dofs + 6 vector representing the generalized bias forces of the robot.
      mask init: same as WBToolboxLibrary/States/GetMeasurement
      mask DialogControl toggleHighlighting Prompt: Toggle Config Block Highlighting
      mask DialogControl toggleHighlighting Callback:
      | [configBlock, ~] = WBToolbox.BlockInitialization(gcb, gcs);
      | 
      | try
      |     if (strcmp(get_param(configBlock,'HiliteAncestors'),'none'))
      |         hilite_system(configBlock,'find');
      |     else
      |         hilite_system(configBlock,'none');
      |     end
      | catch
      |     error('[%s:ShowConfigBlock:Callback] Failed to process config block name: %s',gcb,configBlock);
      | end
      | 
      | clear configBlock
  GetGravityForces : Subsystem  mask(Gravity bias){}
      mask help:
      | This block compute the generalized bias forces due to the gravity
      |
      | Assuming DoFs is the number of internal degrees of freedom of the robot:
      |
      | Input:
      |   - Base pose: 4x4 matrix representing the homogenous transformation between the base frame and the world frame.
      |   - Joint configuration: Vector of size DoFs, representing the configuration of the joints.
      |
      | Output:
      |   - Gravity: a DoFs + 6 vector representing the torques due to the gravity.
      mask init: same as WBToolboxLibrary/States/GetMeasurement
      mask DialogControl toggleHighlighting Prompt: Toggle Config Block Highlighting
      mask DialogControl toggleHighlighting Callback:
      | [configBlock, ~] = WBToolbox.BlockInitialization(gcb, gcs);
      | 
      | try
      |     if (strcmp(get_param(configBlock,'HiliteAncestors'),'none'))
      |         hilite_system(configBlock,'find');
      |     else
      |         hilite_system(configBlock,'none');
      |     end
      | catch
      |     error('[%s:ShowConfigBlock:Callback] Failed to process config block name: %s',gcb,configBlock);
      | end
      | 
      | clear configBlock
  InverseDynamics : S-Function  FunctionName=BlockFactory  Parameters='InverseDynamics','WBToolbox',WBTConfigParameters,configBlockAbsName  SFunctionDeploymentMode=off  EnableBusSupport=off  mask(InverseDynamics){}
      mask help:
      | This block compute the inverse dynamics of the robot.
      |
      | Assuming DoFs is the number of internal degrees of freedom of the robot:
      |
      | Input:
      |   - Base pose: 4x4 matrix representing the homogenous transformation between the base frame and the world frame.
      |   - Joint configuration: Vector of size DoFs, representing the configuration of the joints.
      |   - Base velocity: Vector of size 6 representing the linear and angular velocity of the base frame.
      |   - Joints velocity: Vector of size DoFs, representing the velocity of the joints.
      |   - Base acceleration: Vector of size 6 representing the linear and angular acceleration of the base frame.
      |   - Joints acceleration: Vector of size DoFs, representing the acceleration of the joints.
      |
      | Output:
      |   - Torques: a Dofs + 6 vector representing the corresponding torques required to achive the desired accelerations given the robot state.
      mask init: same as WBToolboxLibrary/States/GetMeasurement
      mask DialogControl toggleHighlighting Prompt: Toggle Config Block Highlighting
      mask DialogControl toggleHighlighting Callback:
      | [configBlock, ~] = WBToolbox.BlockInitialization(gcb, gcs);
      | 
      | try
      |     if (strcmp(get_param(configBlock,'HiliteAncestors'),'none'))
      |         hilite_system(configBlock,'find');
      |     else
      |         hilite_system(configBlock,'none');
      |     end
      | catch
      |     error('[%s:ShowConfigBlock:Callback] Failed to process config block name: %s',gcb,configBlock);
      | end
      | 
      | clear configBlock
      mask Display:
      | port_label('output', 1, 'Torques')
      | 
      | port_label('input', 1, 'Base pose')
      | port_label('input', 2, 'Joints configuration')
      | port_label('input', 3, 'Base velocity')
      | port_label('input', 4, 'Joints velocity')
      | port_label('input', 5, 'Base acceleration')
      | port_label('input', 6, 'Joints acceleration')
  MassMatrix : Subsystem  mask(MassMatrix){}
      mask help:
      | This block retrieves the robot mass matrix.
      |
      | Assuming DoFs is the number of internal degrees of freedom of the robot,
      |
      | Input:
      |   - Base pose: 4x4 matrix representing the homogenous transformation between the base frame and the world frame.
      |   - Joint configuration: Vector of size DoFs, representing the configuration of the joints.
      |
      | Output:
      |   - MassMatrix: a (DoFs + 6) x (DoFs + 6) matrix representing the mass matrix of the robot.
      mask init: same as WBToolboxLibrary/States/GetMeasurement
      mask DialogControl toggleHighlighting Prompt: Toggle Config Block Highlighting
      mask DialogControl toggleHighlighting Callback:
      | [configBlock, ~] = WBToolbox.BlockInitialization(gcb, gcs);
      | 
      | try
      |     if (strcmp(get_param(configBlock,'HiliteAncestors'),'none'))
      |         hilite_system(configBlock,'find');
      |     else
      |         hilite_system(configBlock,'none');
      |     end
      | catch
      |     error('[%s:ShowConfigBlock:Callback] Failed to process config block name: %s',gcb,configBlock);
      | end
      | 
      | clear configBlock
